simulink model "ES101A_DiagcMgr"  (R2013b)
settings: Solver=ode45  StartTime=0.0  StopTime=0.44  RelTol=1e-3
values from neighbouring files (symbols this model uses):
  BrdgVltg = DataDict.IpSignal    [ES101A_DiagcMgr_DataDict.m]
  DEM_CLEAR_PENDING = DataDict.Constant    [ES101A_DiagcMgr_DataDict.m]
  DEM_DTC_GROUP_ALL_DTCS = DataDict.Constant    [ES101A_DiagcMgr_DataDict.m]
  DFTAGICNTR_CNT_U08 = DataDict.Constant    [ES101A_DiagcMgr_DataDict.m]
  DIAGCMGR_NTCINFOSTSTESTFAILD_CNT_U08 = DataDict.Constant    [ES101A_DiagcMgrProxyX_DataDict.m]    (also in ES101A_DiagcMgr_DataDict.m)
  DIAGCMGR_NTCINFOSTSTESTFAILDTHISIGNCYC_CNT_U08 = DataDict.Constant    [ES101A_DiagcMgr_DataDict.m]
  DIAGCMGR_NTCINFOSTSTESTNOTCMPLTHISIGNCYC_CNT_U08 = DataDict.Constant    [ES101A_DiagcMgrProxyX_DataDict.m]    (also in ES101A_DiagcMgr_DataDict.m)
  DiagcMgrFltResp = DataDict.Calibration    [ES101A_DiagcMgrProxyX_DataDict.m]    (also in ES101A_DiagcMgr_DataDict.m)
  DiagcMgrNtcFltAry = DataDict.NVM    [ES101A_DiagcMgr_DataDict.m]
  DIAGCSTSCTRLDSHTDWNFLTPRSNT_CNT_U16 = DataDict.Constant    [ES101A_DiagcMgr_DataDict.m]
  DIAGCSTSDFTHWAG_CNT_U16 = DataDict.Constant    [ES101A_DiagcMgr_DataDict.m]
  DIAGCSTSDFTHWAGSERLCOMEXPRTVAL_CNT_U16 = DataDict.Constant    [ES101A_DiagcMgr_DataDict.m]
  DIAGCSTSDFTVEHSPD_CNT_U16 = DataDict.Constant    [ES101A_DiagcMgr_DataDict.m]
  DIAGCSTSININVAL_CNT_U16 = DataDict.Constant    [ES101A_DiagcMgrProxyX_DataDict.m]    (also in ES101A_DiagcMgr_DataDict.m)
  DIAGCSTSIVTR1INACTV_CNT_U16 = DataDict.Constant    [ES101A_DiagcMgr_DataDict.m]
  DIAGCSTSIVTR2INACTV_CNT_U16 = DataDict.Constant    [ES101A_DiagcMgr_DataDict.m]
  DIAGCSTSLIMDTPRFMNC_CNT_U16 = DataDict.Constant    [ES101A_DiagcMgr_DataDict.m]
  DIAGCSTSRAMPTOZEROFLTPRSNT_CNT_U16 = DataDict.Constant    [ES101A_DiagcMgr_DataDict.m]
  DIAGCSTSWHLIMBREJCTNDI_CNT_U16 = DataDict.Constant    [ES101A_DiagcMgr_DataDict.m]
  DTCIDXSTSFAIL_CNT_U08 = DataDict.Constant    [ES101A_DiagcMgr_DataDict.m]
  DTCIDXSTSNONTC_CNT_U08 = DataDict.Constant    [ES101A_DiagcMgr_DataDict.m]
  DTCIDXSTSNORES_CNT_U08 = DataDict.Constant    [ES101A_DiagcMgr_DataDict.m]
  DTCIDXSTSPASS_CNT_U08 = DataDict.Constant    [ES101A_DiagcMgr_DataDict.m]
  DTCIDXSTSUPDCFMD_CNT_U08 = DataDict.Constant    [ES101A_DiagcMgr_DataDict.m]
  ELECGLBPRM_IVTRCNT_CNT_U08 = DataDict.ConfigParam    [ES101A_DiagcMgrProxyX_DataDict.m]    (also in ES101A_DiagcMgr_DataDict.m)
  FLTINJ_DIAGCMGR_DIAGCSTSIVTR1INACTV = DataDict.Constant    [ES101A_DiagcMgr_DataDict.m]
  FLTINJ_DIAGCMGR_DIAGCSTSIVTR2INACTV = DataDict.Constant    [ES101A_DiagcMgr_DataDict.m]
  HwTq = DataDict.IpSignal    [ES101A_DiagcMgr_DataDict.m]
  IgnCntr = DataDict.IpSignal    [ES101A_DiagcMgr_DataDict.m]
  MAXDEBCNTRVAL_CNT_S16 = DataDict.Constant    [ES101A_DiagcMgr_DataDict.m]
  MAXRAMPRATE_ULSPERSEC_F32 = DataDict.Constant    [ES101A_DiagcMgrProxyX_DataDict.m]    (also in ES101A_DiagcMgr_DataDict.m)
  MINDEBCNTRVAL_CNT_S16 = DataDict.Constant    [ES101A_DiagcMgr_DataDict.m]
  MINRAMPRATE_ULSPERSEC_F32 = DataDict.Constant    [ES101A_DiagcMgrProxyX_DataDict.m]    (also in ES101A_DiagcMgr_DataDict.m)
  SCAMOTTQCMDTOONE_ULS_F32 = DataDict.Constant    [ES101A_DiagcMgrProxyX_DataDict.m]    (also in ES101A_DiagcMgr_DataDict.m)
  SCAMOTTQCMDTOZERO_ULS_F32 = DataDict.Constant    [ES101A_DiagcMgrProxyX_DataDict.m]    (also in ES101A_DiagcMgr_DataDict.m)
  SysSt = DataDict.IpSignal    [ES101A_DiagcMgr_DataDict.m]
  VehSpd = DataDict.IpSignal    [ES101A_DiagcMgr_DataDict.m]
undefined symbols (not defined in the file or in its folder): ActvMotTqCmdSca, ActvRampRate, AgiCntr, Dem_DTCFormatType, Dem_DTCOriginType, Dem_EventStatusType, DiagcData, DiagcMgrNtcMap, DiagcSts, DtcEnaMask, EcuT, HistNtcFltAry, MicroDiagcData, MotTq, NtcNr, NtcNrWithResd1, NtcStInfo, ProxySetNtcData, Sts, SysSt1, TOTNROFDTC_CNT_U08
libraries: simulink x149, FloatToFixd x5, NxtrNvM x3
(part 7 of 13)

== system ES101A_DiagcMgr/DiagcMgr/DiagcMgrPwrDwn/Update NtcFltAry and HistFltAry/For Number of NTCs/Check Aging Counter/Update NtcFltAry ==
  NtcMapIdx : Inport
  Sts : Inport  Port=2
  Action Port : ActionPort
  Add : Sum
  Assignment1 : Assignment  IndexMode=Zero-based  IndexOptions=Index vector (port)  Indices=1  OutputSizes=1
  Bus Assignment1 : BusAssignment  AssignedSignals=NtcNr,AgiCntr,Sts
  Constant : Constant  OutDataTypeStr=uint8
  Constant1 : Constant  OutDataTypeStr=uint8
  CopyRight2 : Subsystem  Description=|  mask(Copyright Information){none=on}
      | Copyright info block.                                               
      |                                                                     
      | Place copyright information at the top of every subsystem in design.
      mask prompts: none "No parameters"
      mask help: Place copyright information at the top of every subsystem in design.
      mask Display:
      | NxtrConf = 'Nexteer Confidential';
      | 
      | sys = bdroot; %handle for the current model ("system")
      | first = get_param(sys,'Created');
      | first = first(end-3:end);  %year is last four digits
      | 
      | last = get_param(sys,'LastModifiedDate');
      | if isempty(last)
      |     last = datestr(now,'yyyy');
      | else
      |     last = last(end-3:end);
      | end
      | 
      | if strcmp(first,last)
      |     fprintf('%s -- Copyright %s Nexteer',NxtrConf,first)
      | else
      |     fprintf('%s -- %s%s- %s Nexteer',NxtrConf,char(169),first,last)
      | end
  Data Store Read1 : DataStoreRead  DataStoreName=NtcFltAryIdx  DataStoreElements=NtcFltAryIdx
  Data Store Read2 : DataStoreRead  DataStoreName=NtcFltAryIdx  DataStoreElements=NtcFltAryIdx
  Data Store Read5 : DataStoreRead  DataStoreName=DiagcMgrNtcFltAry  DataStoreElements=DiagcMgrNtcFltAry(:)
  Data Store Write1 : DataStoreWrite  DataStoreName=NtcFltAryIdx
  Data Store Write2 : DataStoreWrite  DataStoreName=DiagcMgrNtcFltAry  DataStoreElements=DiagcMgrNtcFltAry(:)
  Selector : Selector  IndexMode=Zero-based  InputPortWidth=20  IndexOptions=Index vector (port)  Indices=[1 3]  OutputSizes=1
  wires:
  Sts/1 -> Bus Assignment1/4
  Add/1 -> Data Store Write1/1
  Constant/1 -> Add/2
  Data Store Read1/1 -> Add/1
  NtcMapIdx/1 -> Bus Assignment1/2
  Bus Assignment1/1 -> Assignment1/2
  Assignment1/1 -> Data Store Write2/1
  Data Store Read2/1 -> Selector/2, Assignment1/3
  Selector/1 -> Bus Assignment1/1
  Data Store Read5/1 -> Selector/1, Assignment1/1
  Constant1/1 -> Bus Assignment1/3

== system ES101A_DiagcMgr/DiagcMgr/DiagcMgrPwrDwn/Update NtcFltAry and HistFltAry/For Number of NTCs/Default Case/CopyRight2 ==

== system ES101A_DiagcMgr/DiagcMgr/DiagcMgrPwrDwn/Update NtcFltAry and HistFltAry/For Number of NTCs/GetNtcInfoAppIX/CopyRight2 ==

== system ES101A_DiagcMgr/DiagcMgr/ReadNtcFltAry/Update DiagcMgrReadFltInfoAry and HistReadFltAry/For Number of NTCs/Check Aging Counter/CopyRight2 ==

== system ES101A_DiagcMgr/DiagcMgr/ReadNtcFltAry/Update DiagcMgrReadFltInfoAry and HistReadFltAry/For Number of NTCs/Check Aging Counter/Do Nothing ==
  Action Port : ActionPort
  CopyRight2 : Subsystem  Description=|  mask(Copyright Information){none=on}
      | Copyright info block.                                               
      |                                                                     
      | Place copyright information at the top of every subsystem in design.
      mask prompts: none "No parameters"
      mask help: Place copyright information at the top of every subsystem in design.
      mask Display:
      | NxtrConf = 'Nexteer Confidential';
      | 
      | sys = bdroot; %handle for the current model ("system")
      | first = get_param(sys,'Created');
      | first = first(end-3:end);  %year is last four digits
      | 
      | last = get_param(sys,'LastModifiedDate');
      | if isempty(last)
      |     last = datestr(now,'yyyy');
      | else
      |     last = last(end-3:end);
      | end
      | 
      | if strcmp(first,last)
      |     fprintf('%s -- Copyright %s Nexteer',NxtrConf,first)
      | else
      |     fprintf('%s -- %s%s- %s Nexteer',NxtrConf,char(169),first,last)
      | end

== system ES101A_DiagcMgr/DiagcMgr/ReadNtcFltAry/Update DiagcMgrReadFltInfoAry and HistReadFltAry/For Number of NTCs/Check Aging Counter/Update History Fault Array ==
  NtcMapIdx : Inport
  Sts : Inport  Port=2
  AgiCntr : Inport  Port=3
  NtcStInfo : Inport  Port=4
  Action Port : ActionPort
  CopyRight2 : Subsystem  Description=|  mask(Copyright Information){none=on}
      | Copyright info block.                                               
      |                                                                     
      | Place copyright information at the top of every subsystem in design.
      mask prompts: none "No parameters"
      mask help: Place copyright information at the top of every subsystem in design.
      mask Display:
      | NxtrConf = 'Nexteer Confidential';
      | 
      | sys = bdroot; %handle for the current model ("system")
      | first = get_param(sys,'Created');
      | first = first(end-3:end);  %year is last four digits
      | 
      | last = get_param(sys,'LastModifiedDate');
      | if isempty(last)
      |     last = datestr(now,'yyyy');
      | else
      |     last = last(end-3:end);
      | end
      | 
      | if strcmp(first,last)
      |     fprintf('%s -- Copyright %s Nexteer',NxtrConf,first)
      | else
      |     fprintf('%s -- %s%s- %s Nexteer',NxtrConf,char(169),first,last)
      | end
  Data Store Read3 : DataStoreRead  DataStoreName=HistReadFltAryIdx
  If : If  IfExpression=u1 < 20  ShowElse=off
  If Action Subsystem : Subsystem  TreatAsAtomicUnit=on
  wires:
  If/1 -> If Action Subsystem/Action
  Data Store Read3/1 -> If/1
  Sts/1 -> If Action Subsystem/2(Sts)
  AgiCntr/1 -> If Action Subsystem/3(AgiCntr)
  NtcMapIdx/1 -> If Action Subsystem/1(NtcMapIdx)
  NtcStInfo/1 -> If Action Subsystem/4(NtcStInfo)

== system ES101A_DiagcMgr/DiagcMgr/ReadNtcFltAry/Update DiagcMgrReadFltInfoAry and HistReadFltAry/For Number of NTCs/Check Aging Counter/Update NtcFltAry ==
  NtcMapIdx : Inport
  NtcSts : Inport  Port=2
  NtcStInfo : Inport  Port=3
  Action Port : ActionPort
  Add : Sum
  Assignment1 : Assignment  IndexMode=Zero-based  IndexOptions=Index vector (port)  Indices=1  OutputSizes=1
  Bus Assignment3 : BusAssignment  AssignedSignals=NtcNr,AgiCntr,Sts,NtcStInfo
  Constant : Constant  OutDataTypeStr=uint8
  Constant1 : Constant  Value=0  OutDataTypeStr=uint8
  CopyRight2 : Subsystem  Description=|  mask(Copyright Information){none=on}
      | Copyright info block.                                               
      |                                                                     
      | Place copyright information at the top of every subsystem in design.
      mask prompts: none "No parameters"
      mask help: Place copyright information at the top of every subsystem in design.
      mask Display:
      | NxtrConf = 'Nexteer Confidential';
      | 
      | sys = bdroot; %handle for the current model ("system")
      | first = get_param(sys,'Created');
      | first = first(end-3:end);  %year is last four digits
      | 
      | last = get_param(sys,'LastModifiedDate');
      | if isempty(last)
      |     last = datestr(now,'yyyy');
      | else
      |     last = last(end-3:end);
      | end
      | 
      | if strcmp(first,last)
      |     fprintf('%s -- Copyright %s Nexteer',NxtrConf,first)
      | else
      |     fprintf('%s -- %s%s- %s Nexteer',NxtrConf,char(169),first,last)
      | end
  Data Store Read1 : DataStoreRead  DataStoreName=ReadFltInfoIdx
  Data Store Read2 : DataStoreRead  DataStoreName=ReadFltInfoIdx
  Data Store Read5 : DataStoreRead  DataStoreName=DiagcMgrReadFltInfoAry
  Data Store Write1 : DataStoreWrite  DataStoreName=ReadFltInfoIdx
  Data Store Write2 : DataStoreWrite  DataStoreName=DiagcMgrReadFltInfoAry
  Selector : Selector  IndexMode=Zero-based  InputPortWidth=20  IndexOptions=Index vector (port)  Indices=[1 3]  OutputSizes=1
  wires:
  NtcSts/1 -> Bus Assignment3/4
  Add/1 -> Data Store Write1/1
  Constant/1 -> Add/2
  Data Store Read1/1 -> Add/1
  Bus Assignment3/1 -> Assignment1/2
  Assignment1/1 -> Data Store Write2/1
  Data Store Read2/1 -> Selector/2, Assignment1/3
  Selector/1 -> Bus Assignment3/1
  Data Store Read5/1 -> Selector/1, Assignment1/1
  Constant1/1 -> Bus Assignment3/3
  NtcStInfo/1 -> Bus Assignment3/5
  NtcMapIdx/1 -> Bus Assignment3/2

== system ES101A_DiagcMgr/DiagcMgr/ReadNtcFltAry/Update DiagcMgrReadFltInfoAry and HistReadFltAry/For Number of NTCs/Default Case/CopyRight2 ==

== system ES101A_DiagcMgr/DiagcMgr/ReadNtcFltAry/Update DiagcMgrReadFltInfoAry and HistReadFltAry/For Number of NTCs/GetNtcInfoAppIX/CopyRight2 ==

== system ES101A_DiagcMgr/DiagcMgr/ReadNtcInfoAndDebCntr/ApplX/Debounced/GetNtcDebCntrApplX/CopyRight2 ==

== system ES101A_DiagcMgr/DiagcMgr/SetNtcStsCore/NtcNr is Valid/Diagnostics Not Inhibited/NtcEnabled/CopyRight2 ==

== system ES101A_DiagcMgr/DiagcMgr/SetNtcStsCore/NtcNr is Valid/Diagnostics Not Inhibited/NtcEnabled/Else ==
  Action Port : ActionPort  ActionType=else
  CopyRight2 : Subsystem  Description=|  mask(Copyright Information){none=on}
      | Copyright info block.                                               
      |                                                                     
      | Place copyright information at the top of every subsystem in design.
      mask prompts: none "No parameters"
      mask help: Place copyright information at the top of every subsystem in design.
      mask Display:
      | NxtrConf = 'Nexteer Confidential';
      | 
      | sys = bdroot; %handle for the current model ("system")
      | first = get_param(sys,'Created');
      | first = first(end-3:end);  %year is last four digits
      | 
      | last = get_param(sys,'LastModifiedDate');
      | if isempty(last)
      |     last = datestr(now,'yyyy');
      | else
      |     last = last(end-3:end);
      | end
      | 
      | if strcmp(first,last)
      |     fprintf('%s -- Copyright %s Nexteer',NxtrConf,first)
      | else
      |     fprintf('%s -- %s%s- %s Nexteer',NxtrConf,char(169),first,last)
      | end
  E_NOT_OK : Constant  OutDataTypeStr=uint8
  SetNtcSts_StdRtn : Outport
  wires:
  E_NOT_OK/1 -> SetNtcSts_StdRtn/1

== system ES101A_DiagcMgr/DiagcMgr/SetNtcStsCore/NtcNr is Valid/Diagnostics Not Inhibited/NtcEnabled/NTCSTS_FAILD ==
  NtcNr_ArgIn : Inport
  NtcStInfo_ArgIn : Inport  Port=2
  DiagcData_ArgIn : Inport  Port=3
  ProxySetNtcData_ArgIn : Inport  Port=4
  NtcInfo_ArgIn : Inport  Port=5
  SnapshotDataBus : Inport  Port=6
  Action Port : ActionPort  ActionType=elseif
  CopyRight2 : Subsystem  Description=|  mask(Copyright Information){none=on}
      | Copyright info block.                                               
      |                                                                     
      | Place copyright information at the top of every subsystem in design.
      mask prompts: none "No parameters"
      mask help: Place copyright information at the top of every subsystem in design.
      mask Display:
      | NxtrConf = 'Nexteer Confidential';
      | 
      | sys = bdroot; %handle for the current model ("system")
      | first = get_param(sys,'Created');
      | first = first(end-3:end);  %year is last four digits
      | 
      | last = get_param(sys,'LastModifiedDate');
      | if isempty(last)
      |     last = datestr(now,'yyyy');
      | else
      |     last = last(end-3:end);
      | end
      | 
      | if strcmp(first,last)
      |     fprintf('%s -- Copyright %s Nexteer',NxtrConf,first)
      | else
      |     fprintf('%s -- %s%s- %s Nexteer',NxtrConf,char(169),first,last)
      | end
  E_OK : Constant  Value=0  OutDataTypeStr=uint8
  "Update ISO Bits, Parameter Byte and AgiCntr " : Subsystem  RequirementInfo={} %GIDa_0972a75e_8fce_4abf_9038_8b61dadf0b99
  NtcInfo_ArgOut : Outport
  DiagcData_ArgOut : Outport  Port=2
  ProxySetNtcData_ArgOut : Outport  Port=3
  SetNtcSts_StdRtn : Outport  Port=4
  NtcInfoDebCntr_ArgOut : Outport  Port=5
  wires:
  NtcStInfo_ArgIn/1 -> "Update ISO Bits, Parameter Byte and AgiCntr "/2(NtcStInfo_ArgIn)
  "Update ISO Bits, Parameter Byte and AgiCntr "/1("NtcInfo_ArgOut ") -> NtcInfo_ArgOut/1
  NtcNr_ArgIn/1 -> "Update ISO Bits, Parameter Byte and AgiCntr "/1(NtcNr_ArgIn)
  DiagcData_ArgIn/1 -> "Update ISO Bits, Parameter Byte and AgiCntr "/3(DiagcData_ArgIn)
  ProxySetNtcData_ArgIn/1 -> "Update ISO Bits, Parameter Byte and AgiCntr "/4(ProxySetNtcData_ArgIn)
  NtcInfo_ArgIn/1 -> "Update ISO Bits, Parameter Byte and AgiCntr "/5(NtcInfo_ArgIn)
  "Update ISO Bits, Parameter Byte and AgiCntr "/3(ProxySetNtcData_ArgOut) -> ProxySetNtcData_ArgOut/1
  "Update ISO Bits, Parameter Byte and AgiCntr "/2(DiagcData_ArgOut) -> DiagcData_ArgOut/1
  E_OK/1 -> SetNtcSts_StdRtn/1
  SnapshotDataBus/1 -> "Update ISO Bits, Parameter Byte and AgiCntr "/6(SnapshotDataBus)
  "Update ISO Bits, Parameter Byte and AgiCntr "/4(NtcInfoDebCntr_ArgOut) -> NtcInfoDebCntr_ArgOut/1

== system ES101A_DiagcMgr/DiagcMgr/SetNtcStsCore/NtcNr is Valid/Diagnostics Not Inhibited/NtcEnabled/NTCSTS_PASSD ==
  NtcNr_ArgIn : Inport
  NtcInfo_ArgIn : Inport  Port=2
  Action Port : ActionPort  ActionType=then
  CopyRight2 : Subsystem  Description=|  mask(Copyright Information){none=on}
      | Copyright info block.                                               
      |                                                                     
      | Place copyright information at the top of every subsystem in design.
      mask prompts: none "No parameters"
      mask help: Place copyright information at the top of every subsystem in design.
      mask Display:
      | NxtrConf = 'Nexteer Confidential';
      | 
      | sys = bdroot; %handle for the current model ("system")
      | first = get_param(sys,'Created');
      | first = first(end-3:end);  %year is last four digits
      | 
      | last = get_param(sys,'LastModifiedDate');
      | if isempty(last)
      |     last = datestr(now,'yyyy');
      | else
      |     last = last(end-3:end);
      | end
      | 
      | if strcmp(first,last)
      |     fprintf('%s -- Copyright %s Nexteer',NxtrConf,first)
      | else
      |     fprintf('%s -- %s%s- %s Nexteer',NxtrConf,char(169),first,last)
      | end
  E_OK : Constant  Value=0  OutDataTypeStr=uint8
  "Update NtcInfoSts " : Subsystem  RequirementInfo="{'linktype_rmi_doors' '0000c474 (/ESG Group/FDD Module Requirements/EA4 Specific/ES101A_DiagcMgr)' '#ES101A_237' 'true' 'REQ:  ES101A_237' '' ; 'linktype_rmi_doors' '0000c474 (/ESG Group/FDD Module Requirements/EA4 Specific/ES101A_DiagcMgr)' '#ES101A_193' 'true' 'REQ:  ES101A_193' '' ; 'linktype_rmi_doors' '0000c474 (/ESG Group/FDD Module Requirements/EA4 Specific/ES101A_DiagcMgr)' '#ES101A_253' 'true' 'REQ:  ES101A_253' '' ; 'linktype_rmi_doors' '0000c474 (/ESG Group/FDD Module Requirements/EA4 Specific/ES101A_DiagcMgr)' '#ES101A_194' 'true' 'REQ:  ES101A_194' '' ; 'linktype_rmi_doors' '0000c474 (/ESG Group/FDD Module Requirements/EA4 Specific/ES101A_DiagcMgr)' '#ES101A_195' 'true' 'REQ:  ES101A_195' '' } %GIDa_1a6e31a1_b3c2_4f97_a6bd_4683aee25e70"
  "NtcInfo_ArgOut " : Outport
  SetNtcSts_StdRtn : Outport  Port=2
  NtcInfoDebCntr_ArgOut : Outport  Port=3
  wires:
  "Update NtcInfoSts "/1(NtcInfo_ArgOut) -> "NtcInfo_ArgOut "/1
  NtcInfo_ArgIn/1 -> "Update NtcInfoSts "/1(NtcInfo_ArgIn)
  NtcNr_ArgIn/1 -> "Update NtcInfoSts "/2(NtcNr_ArgIn)
  E_OK/1 -> SetNtcSts_StdRtn/1
  "Update NtcInfoSts "/2(NtcInfoDebCntr_ArgOut) -> NtcInfoDebCntr_ArgOut/1

== system ES101A_DiagcMgr/DiagcMgr/SetNtcStsCore/NtcNr is Valid/Diagnostics Not Inhibited/NtcEnabled/NTCSTS_PREFAILD ==
  NtcNr_ArgIn : Inport
  NtcStInfo_ArgIn : Inport  Port=2
  DebStep_ArgIn : Inport  Port=3
  DiagcData_ArgIn : Inport  Port=4
  ProxySetNtcData_ArgIn : Inport  Port=5
  NtcInfo_ArgIn : Inport  Port=6
  NtcInfoDebCntr_ArgIn : Inport  Port=7
  SnapshotDataBus : Inport  Port=8
  Action Port : ActionPort  ActionType=elseif
  CopyRight2 : Subsystem  Description=|  mask(Copyright Information){none=on}
      | Copyright info block.                                               
      |                                                                     
      | Place copyright information at the top of every subsystem in design.
      mask prompts: none "No parameters"
      mask help: Place copyright information at the top of every subsystem in design.
      mask Display:
      | NxtrConf = 'Nexteer Confidential';
      | 
      | sys = bdroot; %handle for the current model ("system")
      | first = get_param(sys,'Created');
      | first = first(end-3:end);  %year is last four digits
      | 
      | last = get_param(sys,'LastModifiedDate');
      | if isempty(last)
      |     last = datestr(now,'yyyy');
      | else
      |     last = last(end-3:end);
      | end
      | 
      | if strcmp(first,last)
      |     fprintf('%s -- Copyright %s Nexteer',NxtrConf,first)
      | else
      |     fprintf('%s -- %s%s- %s Nexteer',NxtrConf,char(169),first,last)
      | end
  E_OK : Constant  Value=0  OutDataTypeStr=uint8
  "Update NtcInfoSts, DebCntr and Process RampRate" : Subsystem  RequirementInfo="{'linktype_rmi_doors' '0000c474 (/ESG Group/FDD Module Requirements/EA4 Specific/ES101A_DiagcMgr)' '#ES101A_271' 'true' 'REQ:  ES101A_271' '' ; 'linktype_rmi_doors' '0000c474 (/ESG Group/FDD Module Requirements/EA4 Specific/ES101A_DiagcMgr)' '#ES101A_275' 'true' 'REQ:  ES101A_275' '' ; 'linktype_rmi_doors' '0000c474 (/ESG Group/FDD Module Requirements/EA4 Specific/ES101A_DiagcMgr)' '#ES101A_277' 'true' 'REQ:  ES101A_277' '' } %GIDa_7d1c32b8_1a99_4692_8d53_85042ca45bd2"
  NtcInfo_ArgOut : Outport
  NtcInfoDebCntr_ArgOut : Outport  Port=2
  DiagcData_ArgOut : Outport  Port=3
  ProxySetNtcData_ArgOut : Outport  Port=4
  SetNtcSts_StdRtn : Outport  Port=5
  wires:
  DiagcData_ArgIn/1 -> "Update NtcInfoSts, DebCntr and Process RampRate"/5(DiagcData_ArgIn)
  ProxySetNtcData_ArgIn/1 -> "Update NtcInfoSts, DebCntr and Process RampRate"/6(ProxySetNtcData_ArgIn)
  NtcInfo_ArgIn/1 -> "Update NtcInfoSts, DebCntr and Process RampRate"/1(NtcInfo_ArgIn)
  DebStep_ArgIn/1 -> "Update NtcInfoSts, DebCntr and Process RampRate"/2(DebStep_ArgIn)
  NtcStInfo_ArgIn/1 -> "Update NtcInfoSts, DebCntr and Process RampRate"/3(NtcStInfo_ArgIn)
  NtcNr_ArgIn/1 -> "Update NtcInfoSts, DebCntr and Process RampRate"/4(NtcNr_ArgIn)
  "Update NtcInfoSts, DebCntr and Process RampRate"/2(DiagcData_ArgOut) -> DiagcData_ArgOut/1
  "Update NtcInfoSts, DebCntr and Process RampRate"/4(ProxySetNtcData_ArgOut) -> ProxySetNtcData_ArgOut/1
  NtcInfoDebCntr_ArgIn/1 -> "Update NtcInfoSts, DebCntr and Process RampRate"/7(NtcInfoDebCntr_ArgIn)
  "Update NtcInfoSts, DebCntr and Process RampRate"/1(NtcInfo_ArgOut) -> NtcInfo_ArgOut/1
  "Update NtcInfoSts, DebCntr and Process RampRate"/3(NtcInfoDebCntr_ArgOut) -> NtcInfoDebCntr_ArgOut/1
  E_OK/1 -> SetNtcSts_StdRtn/1
  SnapshotDataBus/1 -> "Update NtcInfoSts, DebCntr and Process RampRate"/8(SnapshotDataBus)

== system ES101A_DiagcMgr/DiagcMgr/SetNtcStsCore/NtcNr is Valid/Diagnostics Not Inhibited/NtcEnabled/NTCSTS_PREPASSD ==
  NtcNr_ArgIn : Inport
  DebStep_ArgIn : Inport  Port=2
  NtcInfo_ArgIn : Inport  Port=3
  NtcInfoDebCntr_ArgIn : Inport  Port=4
  Action Port : ActionPort  ActionType=elseif
  CopyRight2 : Subsystem  Description=|  mask(Copyright Information){none=on}
      | Copyright info block.                                               
      |                                                                     
      | Place copyright information at the top of every subsystem in design.
      mask prompts: none "No parameters"
      mask help: Place copyright information at the top of every subsystem in design.
      mask Display:
      | NxtrConf = 'Nexteer Confidential';
      | 
      | sys = bdroot; %handle for the current model ("system")
      | first = get_param(sys,'Created');
      | first = first(end-3:end);  %year is last four digits
      | 
      | last = get_param(sys,'LastModifiedDate');
      | if isempty(last)
      |     last = datestr(now,'yyyy');
      | else
      |     last = last(end-3:end);
      | end
      | 
      | if strcmp(first,last)
      |     fprintf('%s -- Copyright %s Nexteer',NxtrConf,first)
      | else
      |     fprintf('%s -- %s%s- %s Nexteer',NxtrConf,char(169),first,last)
      | end
  E_OK : Constant  Value=0  OutDataTypeStr=uint8
  Update NtcInfoSts : Subsystem  RequirementInfo={} %GIDa_9aed3398_88be_4c57_a651_a29afef92a4a
  NtcInfo_ArgOut : Outport
  NtcInfoDebCntr_ArgOut : Outport  Port=2
  SetNtcSts_StdRtn : Outport  Port=3
  wires:
  DebStep_ArgIn/1 -> Update NtcInfoSts/2(DebStep_ArgIn)
  Update NtcInfoSts/1(NtcInfo_ArgOut) -> NtcInfo_ArgOut/1
  NtcNr_ArgIn/1 -> Update NtcInfoSts/1(NtcNr_ArgIn)
  NtcInfo_ArgIn/1 -> Update NtcInfoSts/3(NtcInfo_ArgIn)
  NtcInfoDebCntr_ArgIn/1 -> Update NtcInfoSts/4(NtcInfoDebCntr_ArgIn)
  Update NtcInfoSts/2(NtcInfoDebCntr_ArgOut) -> NtcInfoDebCntr_ArgOut/1
  E_OK/1 -> SetNtcSts_StdRtn/1

== system ES101A_DiagcMgr/DiagcMgr/SetNtcStsCore/NtcNr is Valid/Diagnostics Not Inhibited/NtcNotEnabled/CopyRight2 ==

== system ES101A_DiagcMgr/DiagcMgr/DiagcMgrIninCore/Initialize the NtcInfo Array/Update the ISO bits of each NTC/Start Initialization/If Action Subsystem/Clear: DIAGCMGR_NTCINFOSTSTESTFAILDTHISIGNCYC_CNT_U08 ==
  In2 : Inport
  In1 : Inport  Port=2
  Bitwise Operator : simulink/Logic and Bit Operations/Bitwise Operator  logicop=NOT  UseBitMask=off  BitMask=bin2dec('11011001')  BitMaskRealWorld=Stored Integer
  Bitwise Operator1 : simulink/Logic and Bit Operations/Bitwise Operator  logicop=AND  UseBitMask=off  NumInputPorts=2  BitMask=bin2dec('11011001')  BitMaskRealWorld=Stored Integer
  Out1 : Outport
  wires:
  Bitwise Operator1/1 -> Out1/1
  In2/1 -> Bitwise Operator1/1
  In1/1 -> Bitwise Operator/1
  Bitwise Operator/1 -> Bitwise Operator1/2

== system ES101A_DiagcMgr/DiagcMgr/DiagcMgrIninCore/Initialize the NtcInfo Array/Update the ISO bits of each NTC/Start Initialization/If Action Subsystem/CopyRight2 ==

== system ES101A_DiagcMgr/DiagcMgr/DiagcMgrIninCore/Initialize the NtcInfo Array/Update the ISO bits of each NTC/Start Initialization/If Action Subsystem1/CopyRight2 ==

== system ES101A_DiagcMgr/DiagcMgr/DiagcMgrIninCore/Update NtcInfoAry From NvM/Update NtcInfoAry/Update NtcInfoAry Aging Counter And Confirmed Bit/If Action/Subsystem ==
  AgiCntr_ArgIn : Inport
  NtcNr : Inport  Port=2
  Sts : Inport  Port=3
  NtcInfoAry_ArgIn : Inport  Port=4
  Action Port : ActionPort  ActionType=then
  0 < AgingCntr < 64 : Subsystem  TreatAsAtomicUnit=on
  AgingCntr >= 64 Do Nothing : Subsystem  TreatAsAtomicUnit=on
  If : If  IfExpression=u1 > 0 & u1 <= 64
  NtcInfoAry_ArgOut : Outport
  wires:
  If/2 -> AgingCntr >= 64 Do Nothing/Action
  If/1 -> 0 < AgingCntr < 64/Action
  NtcNr/1 -> 0 < AgingCntr < 64/1(NtcNr)
  Sts/1 -> 0 < AgingCntr < 64/3("Sts ")
  AgiCntr_ArgIn/1 -> 0 < AgingCntr < 64/2(AgiCntr), If/1
  NtcInfoAry_ArgIn/1 -> 0 < AgingCntr < 64/4(NtcInfoAry_ArgIn)
  0 < AgingCntr < 64/1(NtcInfoAry_ArgOut) -> NtcInfoAry_ArgOut/1

== system ES101A_DiagcMgr/DiagcMgr/DiagcMgrPer2/Clear All DTCs/Call DEM & Update DtcIdxPrevSts/Update DtcIdxPrevSts and PrevClrDtcFlg/Clear All DTCs/CopyRight2 ==

== system ES101A_DiagcMgr/DiagcMgr/DiagcMgrPer2/Clear All DTCs/Call DEM & Update DtcIdxPrevSts/Update DtcIdxPrevSts and PrevClrDtcFlg/Clear All DTCs/For All DTC Indices ==
  DtcIdx : Inport
  Assignment : Assignment  IndexMode=Zero-based  IndexOptions=Starting index (port)  Indices=1  OutputSizes=1
  CopyRight2 : Subsystem  Description=|  mask(Copyright Information){none=on}
      | Copyright info block.                                               
      |                                                                     
      | Place copyright information at the top of every subsystem in design.
      mask prompts: none "No parameters"
      mask help: Place copyright information at the top of every subsystem in design.
      mask Display:
      | NxtrConf = 'Nexteer Confidential';
      | 
      | sys = bdroot; %handle for the current model ("system")
      | first = get_param(sys,'Created');
      | first = first(end-3:end);  %year is last four digits
      | 
      | last = get_param(sys,'LastModifiedDate');
      | if isempty(last)
      |     last = datestr(now,'yyyy');
      | else
      |     last = last(end-3:end);
      | end
      | 
      | if strcmp(first,last)
      |     fprintf('%s -- Copyright %s Nexteer',NxtrConf,first)
      | else
      |     fprintf('%s -- %s%s- %s Nexteer',NxtrConf,char(169),first,last)
      | end
  Data Store Read : DataStoreRead  DataStoreName=DtcIdxPrevSts
  Data Store Write : DataStoreWrite  DataStoreName=DtcIdxPrevSts
  No Res : Constant  Value=DTCIDXSTSNORES_CNT_U08
  wires:
  No Res/1 -> Assignment/2
  DtcIdx/1 -> Assignment/3
  Assignment/1 -> Data Store Write/1
  Data Store Read/1 -> Assignment/1

== system ES101A_DiagcMgr/DiagcMgr/DiagcMgrPer2/Normal Periodic Processing/For All DTCs/For Each DTC/Check If DTC Status has Changed/CopyRight2 ==

== system ES101A_DiagcMgr/DiagcMgr/DiagcMgrPer2/Normal Periodic Processing/For All DTCs/For Each DTC/Check If DTC Status has Changed/DTC Status Changed OR DTC Update NOT Confirmed ==
  DtcIdx : Inport
  Action Port : ActionPort
  CopyRight2 : Subsystem  Description=|  mask(Copyright Information){none=on}
      | Copyright info block.                                               
      |                                                                     
      | Place copyright information at the top of every subsystem in design.
      mask prompts: none "No parameters"
      mask help: Place copyright information at the top of every subsystem in design.
      mask Display:
      | NxtrConf = 'Nexteer Confidential';
      | 
      | sys = bdroot; %handle for the current model ("system")
      | first = get_param(sys,'Created');
      | first = first(end-3:end);  %year is last four digits
      | 
      | last = get_param(sys,'LastModifiedDate');
      | if isempty(last)
      |     last = datestr(now,'yyyy');
      | else
      |     last = last(end-3:end);
      | end
      | 
      | if strcmp(first,last)
      |     fprintf('%s -- Copyright %s Nexteer',NxtrConf,first)
      | else
      |     fprintf('%s -- %s%s- %s Nexteer',NxtrConf,char(169),first,last)
      | end
  Data Store Read1 : DataStoreRead  DataStoreName=DtcIdxCurrSts
  Update DTC Index Previous Status with DTC Index Current Status : Subsystem  Priority=1
      settings: AttributesFormatString=Priority = %<Priority>
  Update DTC Status : Subsystem  Priority=2  TreatAsAtomicUnit=on
      settings: AttributesFormatString=Priority = %<Priority>
  wires:
  Data Store Read1/1 -> Update DTC Status/1(DtcIdxCurrSts)
  DtcIdx/1 -> Update DTC Status/2(DtcIdx), Update DTC Index Previous Status with DTC Index Current Status/1(DtcIdx)

== system ES101A_DiagcMgr/DiagcMgr/DiagcMgrPer2/Normal Periodic Processing/For All NTCs/For Each NTC/DoNothing/CopyRight2 ==

== system ES101A_DiagcMgr/DiagcMgr/DiagcMgrPer2/Normal Periodic Processing/For All NTCs/For Each NTC/GetNtcInfoAppIX/CopyRight2 ==

== system ES101A_DiagcMgr/DiagcMgr/DiagcMgrPer2/Normal Periodic Processing/For All NTCs/For Each NTC/Update DTC Status/CopyRight2 ==

== system ES101A_DiagcMgr/DiagcMgr/DiagcMgrPer2/Normal Periodic Processing/For All NTCs/For Each NTC/Update DTC Status/NTC Enabled ==
  DtcIdx : Inport
  NtcSts : Inport  Port=2
  Action Port : ActionPort
  Compare to Zero2 : simulink/Logic and Bit Operations/Compare To Zero  relop=~=  OutDataTypeStr=boolean
  Compare to Zero3 : simulink/Logic and Bit Operations/Compare To Zero  relop=~=  OutDataTypeStr=boolean
  CopyRight2 : Subsystem  Description=|  mask(Copyright Information){none=on}
      | Copyright info block.                                               
      |                                                                     
      | Place copyright information at the top of every subsystem in design.
      mask prompts: none "No parameters"
      mask help: Place copyright information at the top of every subsystem in design.
      mask Display:
      | NxtrConf = 'Nexteer Confidential';
      | 
      | sys = bdroot; %handle for the current model ("system")
      | first = get_param(sys,'Created');
      | first = first(end-3:end);  %year is last four digits
      | 
      | last = get_param(sys,'LastModifiedDate');
      | if isempty(last)
      |     last = datestr(now,'yyyy');
      | else
      |     last = last(end-3:end);
      | end
      | 
      | if strcmp(first,last)
      |     fprintf('%s -- Copyright %s Nexteer',NxtrConf,first)
      | else
      |     fprintf('%s -- %s%s- %s Nexteer',NxtrConf,char(169),first,last)
      | end
  DIAGCMGR_NTCINFOSTSTESTFAILD_CNT_U08 : simulink/Logic and Bit Operations/Bitwise Operator  logicop=AND  UseBitMask=on  BitMask=DIAGCMGR_NTCINFOSTSTESTFAILD_CNT_U08  BitMaskRealWorld=Stored Integer
  DIAGCMGR_NTCINFOSTSTESTNOTCMPLTHISIGNCYC_CNT_U08 : simulink/Logic and Bit Operations/Bitwise Operator  logicop=AND  UseBitMask=on  BitMask=DIAGCMGR_NTCINFOSTSTESTNOTCMPLTHISIGNCYC_CNT_U08  BitMaskRealWorld=Stored Integer
  DTC Fail : Subsystem  TreatAsAtomicUnit=on
  DTC NoRes : Subsystem  TreatAsAtomicUnit=on
  DTC Pass : Subsystem  TreatAsAtomicUnit=on
  Data Store Read : DataStoreRead  DataStoreName=DtcIdxCurrSts
  Do Nothing : Subsystem  TreatAsAtomicUnit=on
  If : If  NumInputs=2  IfExpression=(u2 == 2)|(u1 == 2)  ElseIfExpressions=(u2 == 0), ((u2 == 1) & ((u1 == 3)|(u1 == 1)))
  If1 : If  NumInputs=2  IfExpression=u1 == 1  ElseIfExpressions=u2 == 0
  Merge : Merge  Inputs=3
  SIGQLFR_FAILD : Subsystem  TreatAsAtomicUnit=on
  SIGQLFR_NORES : Subsystem  TreatAsAtomicUnit=on
  SIGQLFR_PASSD : Subsystem  TreatAsAtomicUnit=on
  Selector1 : Selector  IndexMode=Zero-based  InputPortWidth=512  IndexOptions=Index vector (port)  Indices=[1 3]  OutputSizes=1
  wires:
  NtcSts/1 -> DIAGCMGR_NTCINFOSTSTESTFAILD_CNT_U08/1, DIAGCMGR_NTCINFOSTSTESTNOTCMPLTHISIGNCYC_CNT_U08/1
  DtcIdx/1 -> [DtcIdx], Selector1/2
  Data Store Read/1 -> Selector1/1
  Selector1/1 -> If/1
  DIAGCMGR_NTCINFOSTSTESTNOTCMPLTHISIGNCYC_CNT_U08/1 -> Compare to Zero2/1
  DIAGCMGR_NTCINFOSTSTESTFAILD_CNT_U08/1 -> Compare to Zero3/1
  SIGQLFR_NORES/1(NtcQlfr) -> Merge/1
  SIGQLFR_PASSD/1(NtcQlfr) -> Merge/2
  SIGQLFR_FAILD/1(NtcQlfr) -> Merge/3
  If1/3 -> SIGQLFR_FAILD/Action
  If1/2 -> SIGQLFR_PASSD/Action
  If1/1 -> SIGQLFR_NORES/Action
  Compare to Zero2/1 -> If1/1
  Compare to Zero3/1 -> If1/2
  Merge/1 -> If/2
  If/1 -> DTC Fail/Action
  If/4 -> Do Nothing/Action
  If/3 -> DTC Pass/Action
  If/2 -> DTC NoRes/Action
  [DtcIdx] -> DTC Fail/1(DtcIdx)
  [DtcIdx] -> DTC NoRes/1(DtcIdx)
  [DtcIdx] -> DTC Pass/1(DtcIdx)

== system ES101A_DiagcMgr/DiagcMgr/DiagcMgrPer2/Normal Periodic Processing/For All NTCs/For Each NTC/Update DTC Status/NTC Not Enabled ==
  Action Port : ActionPort
  CopyRight2 : Subsystem  Description=|  mask(Copyright Information){none=on}
      | Copyright info block.                                               
      |                                                                     
      | Place copyright information at the top of every subsystem in design.
      mask prompts: none "No parameters"
      mask help: Place copyright information at the top of every subsystem in design.
      mask Display:
      | NxtrConf = 'Nexteer Confidential';
      | 
      | sys = bdroot; %handle for the current model ("system")
      | first = get_param(sys,'Created');
      | first = first(end-3:end);  %year is last four digits
      | 
      | last = get_param(sys,'LastModifiedDate');
      | if isempty(last)
      |     last = datestr(now,'yyyy');
      | else
      |     last = last(end-3:end);
      | end
      | 
      | if strcmp(first,last)
      |     fprintf('%s -- Copyright %s Nexteer',NxtrConf,first)
      | else
      |     fprintf('%s -- %s%s- %s Nexteer',NxtrConf,char(169),first,last)
      | end

== system ES101A_DiagcMgr/DiagcMgr/DiagcMgrPwrDwn/Update NtcFltAry and HistFltAry/For Number of NTCs/Check Aging Counter/Do Nothing/CopyRight2 ==

== system ES101A_DiagcMgr/DiagcMgr/DiagcMgrPwrDwn/Update NtcFltAry and HistFltAry/For Number of NTCs/Check Aging Counter/Update History Fault Array/CopyRight2 ==

== system ES101A_DiagcMgr/DiagcMgr/DiagcMgrPwrDwn/Update NtcFltAry and HistFltAry/For Number of NTCs/Check Aging Counter/Update History Fault Array/If Action Subsystem ==
  NtcMapIdx : Inport
  Sts : Inport  Port=2
  AgiCntr : Inport  Port=3
  Action Port : ActionPort  ActionType=then
  Add : Sum
  Add1 : Sum
  Assignment1 : Assignment  IndexMode=Zero-based  IndexOptions=Index vector (port)  Indices=1  OutputSizes=1
  Bus Assignment1 : BusAssignment  AssignedSignals=NtcNr,AgiCntr,Sts
  Constant : Constant  OutDataTypeStr=uint8
  Constant1 : Constant  OutDataTypeStr=uint8
  CopyRight2 : Subsystem  Description=|  mask(Copyright Information){none=on}
      | Copyright info block.                                               
      |                                                                     
      | Place copyright information at the top of every subsystem in design.
      mask prompts: none "No parameters"
      mask help: Place copyright information at the top of every subsystem in design.
      mask Display:
      | NxtrConf = 'Nexteer Confidential';
      | 
      | sys = bdroot; %handle for the current model ("system")
      | first = get_param(sys,'Created');
      | first = first(end-3:end);  %year is last four digits
      | 
      | last = get_param(sys,'LastModifiedDate');
      | if isempty(last)
      |     last = datestr(now,'yyyy');
      | else
      |     last = last(end-3:end);
      | end
      | 
      | if strcmp(first,last)
      |     fprintf('%s -- Copyright %s Nexteer',NxtrConf,first)
      | else
      |     fprintf('%s -- %s%s- %s Nexteer',NxtrConf,char(169),first,last)
      | end
  Data Store Read1 : DataStoreRead  DataStoreName=HistFltAryIdx
  Data Store Read2 : DataStoreRead  DataStoreName=HistFltAryIdx  DataStoreElements=HistFltAryIdx
  Data Store Read5 : DataStoreRead  DataStoreName=HistNtcFltAry  DataStoreElements=HistNtcFltAry(:)
  Data Store Write1 : DataStoreWrite  DataStoreName=HistFltAryIdx
  Data Store Write2 : DataStoreWrite  DataStoreName=HistNtcFltAry  DataStoreElements=HistNtcFltAry(:)
  Selector : Selector  IndexMode=Zero-based  InputPortWidth=20  IndexOptions=Index vector (port)  Indices=[1 3]  OutputSizes=1
  wires:
  Sts/1 -> Bus Assignment1/4
  Add/1 -> Data Store Write1/1
  Constant/1 -> Add/2
  Data Store Read1/1 -> Add/1
  NtcMapIdx/1 -> Bus Assignment1/2
  Bus Assignment1/1 -> Assignment1/2
  Assignment1/1 -> Data Store Write2/1
  Data Store Read2/1 -> Selector/2, Assignment1/3
  Selector/1 -> Bus Assignment1/1
  Data Store Read5/1 -> Selector/1, Assignment1/1
  Constant1/1 -> Add1/2
  Add1/1 -> Bus Assignment1/3
  AgiCntr/1 -> Add1/1

== system ES101A_DiagcMgr/DiagcMgr/DiagcMgrPwrDwn/Update NtcFltAry and HistFltAry/For Number of NTCs/Check Aging Counter/Update NtcFltAry/CopyRight2 ==

== system ES101A_DiagcMgr/DiagcMgr/ReadNtcFltAry/Update DiagcMgrReadFltInfoAry and HistReadFltAry/For Number of NTCs/Check Aging Counter/Do Nothing/CopyRight2 ==

== system ES101A_DiagcMgr/DiagcMgr/ReadNtcFltAry/Update DiagcMgrReadFltInfoAry and HistReadFltAry/For Number of NTCs/Check Aging Counter/Update History Fault Array/CopyRight2 ==

== system ES101A_DiagcMgr/DiagcMgr/ReadNtcFltAry/Update DiagcMgrReadFltInfoAry and HistReadFltAry/For Number of NTCs/Check Aging Counter/Update History Fault Array/If Action Subsystem ==
  NtcMapIdx : Inport
  Sts : Inport  Port=2
  AgiCntr : Inport  Port=3
  NtcStInfo : Inport  Port=4
  Action Port : ActionPort
  Add : Sum
  Assignment1 : Assignment  IndexMode=Zero-based  IndexOptions=Index vector (port)  Indices=1  OutputSizes=1
  Bus Assignment1 : BusAssignment  AssignedSignals=NtcNr,AgiCntr,Sts,NtcStInfo
  Constant : Constant  OutDataTypeStr=uint8
  CopyRight2 : Subsystem  Description=|  mask(Copyright Information){none=on}
      | Copyright info block.                                               
      |                                                                     
      | Place copyright information at the top of every subsystem in design.
      mask prompts: none "No parameters"
      mask help: Place copyright information at the top of every subsystem in design.
      mask Display:
      | NxtrConf = 'Nexteer Confidential';
      | 
      | sys = bdroot; %handle for the current model ("system")
      | first = get_param(sys,'Created');
      | first = first(end-3:end);  %year is last four digits
      | 
      | last = get_param(sys,'LastModifiedDate');
      | if isempty(last)
      |     last = datestr(now,'yyyy');
      | else
      |     last = last(end-3:end);
      | end
      | 
      | if strcmp(first,last)
      |     fprintf('%s -- Copyright %s Nexteer',NxtrConf,first)
      | else
      |     fprintf('%s -- %s%s- %s Nexteer',NxtrConf,char(169),first,last)
      | end
  Data Store Read1 : DataStoreRead  DataStoreName=HistReadFltAryIdx
  Data Store Read2 : DataStoreRead  DataStoreName=HistReadFltAryIdx
  Data Store Read5 : DataStoreRead  DataStoreName=HistReadFltAry
  Data Store Write1 : DataStoreWrite  DataStoreName=HistReadFltAryIdx
  Data Store Write2 : DataStoreWrite  DataStoreName=HistReadFltAry
  Selector : Selector  IndexMode=Zero-based  InputPortWidth=20  IndexOptions=Index vector (port)  Indices=[1 3]  OutputSizes=1
  wires:
  Add/1 -> Data Store Write1/1
  Constant/1 -> Add/2
  Data Store Read1/1 -> Add/1
  Assignment1/1 -> Data Store Write2/1
  Data Store Read2/1 -> Selector/2, Assignment1/3
  Data Store Read5/1 -> Selector/1, Assignment1/1
  Bus Assignment1/1 -> Assignment1/2
  Selector/1 -> Bus Assignment1/1
  NtcStInfo/1 -> Bus Assignment1/5
  Sts/1 -> Bus Assignment1/4
  AgiCntr/1 -> Bus Assignment1/3
  NtcMapIdx/1 -> Bus Assignment1/2

== system ES101A_DiagcMgr/DiagcMgr/ReadNtcFltAry/Update DiagcMgrReadFltInfoAry and HistReadFltAry/For Number of NTCs/Check Aging Counter/Update NtcFltAry/CopyRight2 ==

== system ES101A_DiagcMgr/DiagcMgr/SetNtcStsCore/NtcNr is Valid/Diagnostics Not Inhibited/NtcEnabled/Else/CopyRight2 ==

== system ES101A_DiagcMgr/DiagcMgr/SetNtcStsCore/NtcNr is Valid/Diagnostics Not Inhibited/NtcEnabled/NTCSTS_FAILD/CopyRight2 ==

== system ES101A_DiagcMgr/DiagcMgr/SetNtcStsCore/NtcNr is Valid/Diagnostics Not Inhibited/NtcEnabled/NTCSTS_FAILD/Update ISO Bits, Parameter Byte and AgiCntr  ==
  NtcNr_ArgIn : Inport
  NtcStInfo_ArgIn : Inport  Port=2
  DiagcData_ArgIn : Inport  Port=3
  ProxySetNtcData_ArgIn : Inport  Port=4
  NtcInfo_ArgIn : Inport  Port=5
  SnapshotDataBus : Inport  Port=6
  CopyRight2 : Subsystem  Description=|  mask(Copyright Information){none=on}
      | Copyright info block.                                               
      |                                                                     
      | Place copyright information at the top of every subsystem in design.
      mask prompts: none "No parameters"
      mask help: Place copyright information at the top of every subsystem in design.
      mask Display:
      | NxtrConf = 'Nexteer Confidential';
      | 
      | sys = bdroot; %handle for the current model ("system")
      | first = get_param(sys,'Created');
      | first = first(end-3:end);  %year is last four digits
      | 
      | last = get_param(sys,'LastModifiedDate');
      | if isempty(last)
      |     last = datestr(now,'yyyy');
      | else
      |     last = last(end-3:end);
      | end
      | 
      | if strcmp(first,last)
      |     fprintf('%s -- Copyright %s Nexteer',NxtrConf,first)
      | else
      |     fprintf('%s -- %s%s- %s Nexteer',NxtrConf,char(169),first,last)
      | end
  ProcessRampResponse and DiagcSts : Subsystem  RequirementInfo="{'linktype_rmi_doors' '0000c474 (/ESG Group/FDD Module Requirements/EA4 Specific/ES101A_DiagcMgr)' '#ES101A_73' 'true' 'REQ:  ES101A_73' '' ; 'linktype_rmi_doors' '0000c474 (/ESG Group/FDD Module Requirements/EA4 Specific/ES101A_DiagcMgr)' '#ES101A_290' 'true' 'REQ:  ES101A_290' '' } %GIDa_7dbfdcbb_34ae_4403_b066_54eb6ad30830"
  UpdSnpshtData : Subsystem  RequirementInfo="{'linktype_rmi_doors' '0000c474 (/ESG Group/FDD Module Requirements/EA4 Specific/ES101A_DiagcMgr)' '#ES101A_327' 'true' 'REQ:  ES101A_327' '' ; 'linktype_rmi_doors' '0000c474 (/ESG Group/FDD Module Requirements/EA4 Specific/ES101A_DiagcMgr)' '#ES101A_329' 'true' 'REQ:  ES101A_329' '' ; 'linktype_rmi_doors' '0000c474 (/ESG Group/FDD Module Requirements/EA4 Specific/ES101A_DiagcMgr)' '#ES101A_338' 'true' 'REQ:  ES101A_338' '' } %GIDa_dc21e953_fcab_4714_b08c_f0f43d9730bc"
  "Update ISO Bits, Parameter Byte and AgiCntr" : Subsystem  RequirementInfo="{'linktype_rmi_doors' '0000c474 (/ESG Group/FDD Module Requirements/EA4 Specific/ES101A_DiagcMgr)' '#ES101A_169' 'true' 'REQ:  ES101A_169' '' ; 'linktype_rmi_doors' '0000c474 (/ESG Group/FDD Module Requirements/EA4 Specific/ES101A_DiagcMgr)' '#ES101A_189' 'true' 'REQ:  ES101A_189' '' ; 'linktype_rmi_doors' '0000c474 (/ESG Group/FDD Module Requirements/EA4 Specific/ES101A_DiagcMgr)' '#ES101A_251' 'true' 'REQ:  ES101A_251' '' ; 'linktype_rmi_doors' '0000c474 (/ESG Group/FDD Module Requirements/EA4 Specific/ES101A_DiagcMgr)' '#ES101A_190' 'true' 'REQ:  ES101A_190' '' ; 'linktype_rmi_doors' '0000c474 (/ESG Group/FDD Module Requirements/EA4 Specific/ES101A_DiagcMgr)' '#ES101A_191' 'true' 'REQ:  ES101A_191' '' } %GIDa_2758f62f_4863_4c4b_b93f_16a036f6ed6f"
  "NtcInfo_ArgOut " : Outport
  DiagcData_ArgOut : Outport  Port=2
  ProxySetNtcData_ArgOut : Outport  Port=3
  NtcInfoDebCntr_ArgOut : Outport  Port=4
  wires:
  "Update ISO Bits, Parameter Byte and AgiCntr"/1("NtcInfo_ArgOut ") -> "NtcInfo_ArgOut "/1
  DiagcData_ArgIn/1 -> ProcessRampResponse and DiagcSts/2(DiagcData_ArgIn)
  NtcInfo_ArgIn/1 -> "Update ISO Bits, Parameter Byte and AgiCntr"/2(NtcInfo_ArgIn)
  NtcNr_ArgIn/1 -> UpdSnpshtData/1(NtcNr), ProcessRampResponse and DiagcSts/1(NtcNr_ArgIn)
  ProxySetNtcData_ArgIn/1 -> ProcessRampResponse and DiagcSts/3(ProxySetNtcData_ArgIn)
  ProcessRampResponse and DiagcSts/1(DiagcData_ArgOut) -> DiagcData_ArgOut/1
  ProcessRampResponse and DiagcSts/2(ProxySetNtcData_ArgOut) -> ProxySetNtcData_ArgOut/1
  NtcStInfo_ArgIn/1 -> UpdSnpshtData/2(NtcStInfo), "Update ISO Bits, Parameter Byte and AgiCntr"/1(NtcStInfo_ArgIn)
  SnapshotDataBus/1 -> UpdSnpshtData/3(SnapshotDataBus)
  "Update ISO Bits, Parameter Byte and AgiCntr"/2(NtcInfoDebCntr_ArgOut) -> NtcInfoDebCntr_ArgOut/1

== system ES101A_DiagcMgr/DiagcMgr/SetNtcStsCore/NtcNr is Valid/Diagnostics Not Inhibited/NtcEnabled/NTCSTS_PASSD/CopyRight2 ==

== system ES101A_DiagcMgr/DiagcMgr/SetNtcStsCore/NtcNr is Valid/Diagnostics Not Inhibited/NtcEnabled/NTCSTS_PASSD/Update NtcInfoSts  ==
  NtcInfo_ArgIn : Inport
  NtcNr_ArgIn : Inport  Port=2
  " DIAGCMGR_NTCINFOSTSTESTFAILDTHISIGNCYC_CNT_U08" : simulink/Logic and Bit Operations/Bitwise Operator  logicop=AND  UseBitMask=on  BitMask=DIAGCMGR_NTCINFOSTSTESTFAILDTHISIGNCYC_CNT_U08  BitMaskRealWorld=Stored Integer
  Bus Selector : BusSelector  OutputSignals=Sts
  Data Type Conversion : DataTypeConversion  OutDataTypeStr=boolean
  Data Type Conversion1 : DataTypeConversion  OutDataTypeStr=boolean
  Data Type Conversion2 : DataTypeConversion  OutDataTypeStr=uint16
  Do Nothing : Subsystem
  FLTRESPRCVRLFLT_CNT_U32 : simulink/Logic and Bit Operations/Bitwise Operator  logicop=AND  UseBitMask=on  BitMask=FLTRESPRCVRLFLT_CNT_U32  BitMaskRealWorld=Stored Integer
  Fault Response Table : Constant  Value=DiagcMgrFltResp
  If : If  NumInputs=2  IfExpression=(u1 == 1)|(u2 == 0)
  Selector1 : Selector  IndexMode=Zero-based  InputPortWidth=512  IndexOptions=Index vector (port)  Indices=[1 3]  OutputSizes=1
  Update NTC Info's Status Byte : Subsystem
  NtcInfo_ArgOut : Outport
  NtcInfoDebCntr_ArgOut : Outport  Port=2
  wires:
  NtcNr_ArgIn/1 -> Data Type Conversion2/1
  NtcInfo_ArgIn/1 -> Update NTC Info's Status Byte/1(NtcInfo_ArgIn), Bus Selector/1
  Data Type Conversion2/1 -> Selector1/2
  Data Type Conversion1/1 -> If/2
  Update NTC Info's Status Byte/1(NtcInfo_ArgOut) -> NtcInfo_ArgOut/1
  Fault Response Table/1 -> Selector1/1
  " DIAGCMGR_NTCINFOSTSTESTFAILDTHISIGNCYC_CNT_U08"/1 -> Data Type Conversion1/1
  Data Type Conversion/1 -> If/1
  If/1 -> Update NTC Info's Status Byte/Action
  Bus Selector/1 -> " DIAGCMGR_NTCINFOSTSTESTFAILDTHISIGNCYC_CNT_U08"/1  "<Sts>"
  FLTRESPRCVRLFLT_CNT_U32/1 -> Data Type Conversion/1
  Selector1/1 -> FLTRESPRCVRLFLT_CNT_U32/1
  If/2 -> Do Nothing/Action
  Update NTC Info's Status Byte/2(NtcInfoDebCntr_ArgOut) -> NtcInfoDebCntr_ArgOut/1

== system ES101A_DiagcMgr/DiagcMgr/SetNtcStsCore/NtcNr is Valid/Diagnostics Not Inhibited/NtcEnabled/NTCSTS_PREFAILD/CopyRight2 ==
